simulink model "Octocopter2D_06States"  (R2018b)
settings: Solver=VariableStepAuto  StartTime=0.0  StopTime=10  MaxStep=1e-3  RelTol=1e-3
undefined symbols (not defined in the file): Uav
libraries: simulink_extras x3
settings Model: Creator=jeremie  LastModifiedBy=jban039
settings SFSimCC: SimUseLocalCustomCode=off
settings RTWCC: RTWUseLocalCustomCode=off

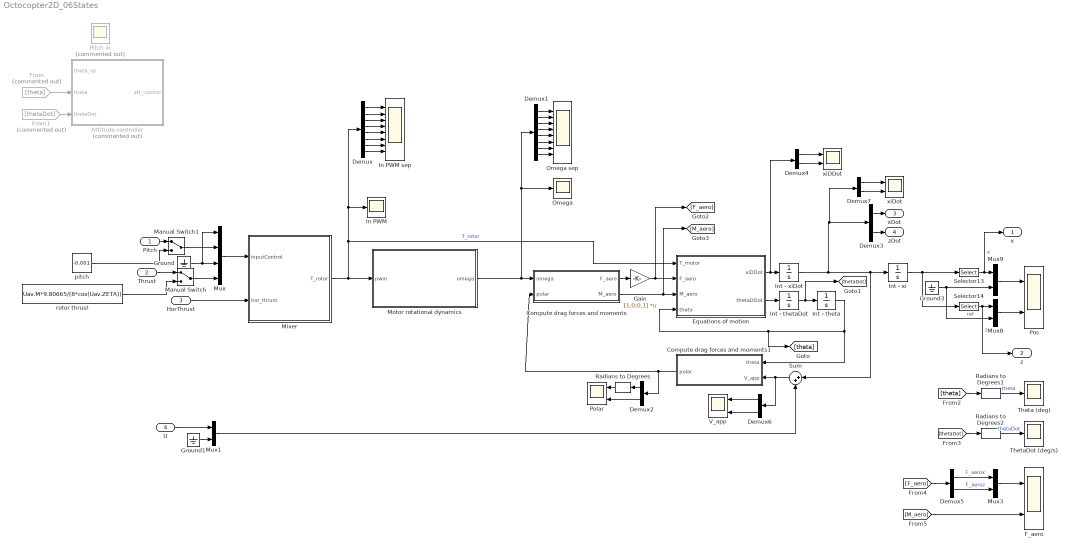
== system Octocopter2D_06States ==
  Pitch : Inport
  Thrust : Inport  Port=2
  HorThrust : Inport  Port=3
  U : Inport  Port=4
  Attitude controller : Subsystem  Commented=on
  Compute drag forces and moments : MATLAB Function  TreatAsAtomicUnit=on
  Compute drag forces and moments1 : MATLAB Function  TreatAsAtomicUnit=on
  Demux : Demux  Outputs=8
  Demux1 : Demux  Outputs=8
  Demux{2..7} (6 alike) : Demux  Outputs=2
  Equations of motion : MATLAB Function  TreatAsAtomicUnit=on
  F_aero : Scope  NumInputPorts=2
  From : From  Commented=on  GotoTag=theta
  From1 : From  Commented=on  GotoTag=thetaDot
  Gain : Gain  Gain=[1,0;0,1]  Multiplication=Matrix(K*u)
  Ground : Ground
  Ground1 : Ground
  Ground3 : Ground
  In PWM : Scope
  In PWM sep : Scope  NumInputPorts=8
  Int - theta : Integrator  ContinuousStateAttributes='theta'
  Int - thetaDot : Integrator  ContinuousStateAttributes='thetaDot'
  Int - xi : Integrator  ContinuousStateAttributes={'x','z'}
  Int - xiDot : Integrator  ContinuousStateAttributes={'xDot','zDot'}
  Manual Switch : ManualSwitch
  Manual Switch1 : ManualSwitch
  Mixer : MATLAB Function  TreatAsAtomicUnit=on
  Motor rotational dynamics : MATLAB Function  TreatAsAtomicUnit=on
  Mux : Mux
  Mux{1,3,8..9} (4 alike) : Mux  Inputs=2
  Omega : Scope
  Omega sep : Scope  NumInputPorts=8
  Pitch in : Scope  Commented=on
  Polar : Scope  NumInputPorts=2
  Pos : Scope  NumInputPorts=2
  Radians to Degrees : simulink_extras/Transformations/Radians to Degrees
  Radians to Degrees1 : simulink_extras/Transformations/Radians to Degrees
  Radians to Degrees2 : simulink_extras/Transformations/Radians to Degrees
  Selector13 : Selector  InputPortWidth=2  IndexOptions=Index vector (dialog)  Indices=1  OutputSizes=1
  Selector14 : Selector  InputPortWidth=2  IndexOptions=Index vector (dialog)  Indices=2  OutputSizes=1
  Sum : Sum  Inputs=|++
  Theta (deg) : Scope
  ThetaDot (deg/s) : Scope
  V_app : Scope  NumInputPorts=2
  pitch : Constant  Value=-0.001
  rotor thrust : Constant  Value=Uav.M*9.80665/(8*cos(Uav.ZETA))
  xiDDot : Scope  NumInputPorts=2
  xiDot : Scope  NumInputPorts=2
  x : Outport
  z : Outport  Port=2
  xDot : Outport  Port=3
  zDot : Outport  Port=4
  wires:
  Motor rotational dynamics/1(omega) -> Compute drag forces and moments/1(omega), Omega/1, Demux1/1
  Compute drag forces and moments/1(F_aero) -> Gain/1
  Compute drag forces and moments/2(M_aero) -> Equations of motion/3(M_aero), [M_aero]
  Mixer/1(T_rotor) -> Demux/1, In PWM/1, Equations of motion/1(T_motor), Motor rotational dynamics/1(pwm)  "T_rotor"
  Mux/1 -> Mixer/1(inputControl)
  Ground/1 -> Mux/3, Mux/1
  Manual Switch1/1 -> Mux/2
  Manual Switch/1 -> Mux/4
  Equations of motion/1(xiDDot) -> Demux4/1, Int - xiDot/1
  Equations of motion/2(thetaDDot) -> Int - thetaDot/1
  Int - thetaDot/1 -> [thetaDot], Int - theta/1
  Int - theta/1 -> [theta], Equations of motion/4(theta), Compute drag forces and moments1/1(theta)
  Mux1/1 -> Sum/2
  Sum/1 -> Demux6/1, Compute drag forces and moments1/2(V_app)
  Compute drag forces and moments1/1(polar) -> Demux2/1, Compute drag forces and moments/2(polar)
  Ground3/1 -> Mux8/2, Mux9/2  "ref"
  Selector14/1 -> z/1, Mux8/1  "z"
  Selector13/1 -> x/1, Mux9/1  "x"
  Mux8/1 -> Pos/2
  Mux9/1 -> Pos/1
  Int - xi/1 -> Selector14/1, Selector13/1
  Demux/1 -> In PWM sep/1
  Demux/2 -> In PWM sep/2
  Demux/3 -> In PWM sep/3
  Demux/4 -> In PWM sep/4
  Demux/5 -> In PWM sep/5
  Demux/6 -> In PWM sep/6
  Demux/7 -> In PWM sep/7
  Demux/8 -> In PWM sep/8
  Demux1/8 -> Omega sep/8
  Demux1/7 -> Omega sep/7
  Demux1/6 -> Omega sep/6
  Demux1/5 -> Omega sep/5
  Demux1/4 -> Omega sep/4
  Demux1/3 -> Omega sep/3
  Demux1/2 -> Omega sep/2
  Demux1/1 -> Omega sep/1
  Demux2/2 -> Polar/2
  Demux2/1 -> Radians to Degrees/1
  Radians to Degrees/1 -> Polar/1
  Radians to Degrees1/1 -> Theta (deg)/1  "theta"
  From/1 -> Attitude controller/2(theta)
  From1/1 -> Attitude controller/3(thetaDot)
  HorThrust/1 -> Mixer/2(hor_thrust)
  [theta] -> Radians to Degrees1/1
  Demux3/1 -> xDot/1
  Demux3/2 -> zDot/1
  Demux4/1 -> xiDDot/1
  Demux4/2 -> xiDDot/2
  [thetaDot] -> Radians to Degrees2/1
  Radians to Degrees2/1 -> ThetaDot (deg/s)/1  "thetaDot"
  U/1 -> Mux1/1
  Ground1/1 -> Mux1/2
  Mux3/1 -> F_aero/1
  [M_aero] -> F_aero/2
  Demux5/1 -> Mux3/1  "F_aerox"
  Demux5/2 -> Mux3/2  "F_aeroz"
  [F_aero] -> Demux5/1
  Thrust/1 -> Manual Switch/1
  rotor thrust/1 -> Manual Switch/2
  Pitch/1 -> Manual Switch1/1
  pitch/1 -> Manual Switch1/2
  Demux6/1 -> V_app/1
  Demux6/2 -> V_app/2
  Demux7/2 -> xiDot/2
  Demux7/1 -> xiDot/1
  Int - xiDot/1 -> Demux7/1, Demux3/1, Sum/1, Int - xi/1
  Gain/1 -> Equations of motion/2(F_aero), [F_aero]

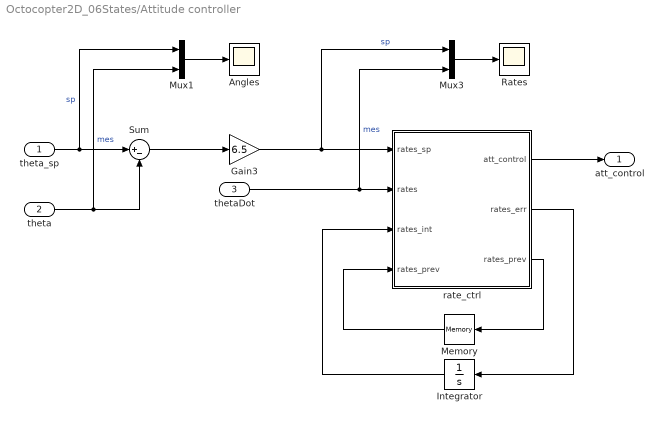
== system Octocopter2D_06States/Attitude controller ==
  theta_sp : Inport
  theta : Inport  Port=2
  thetaDot : Inport  Port=3
  Angles : Scope
  Gain3 : Gain  Gain=6.5
  Integrator : Integrator
  Memory : Memory
  Mux1 : Mux  Inputs=2
  Mux3 : Mux  Inputs=2
  Rates : Scope
  Sum : Sum  Inputs=|+-
  rate_ctrl : MATLAB Function  TreatAsAtomicUnit=on  SystemSampleTime=0.002
  att_control : Outport
  wires:
  rate_ctrl/2(rates_err) -> Integrator/1
  rate_ctrl/3(rates_prev) -> Memory/1
  Integrator/1 -> rate_ctrl/3(rates_int)
  rate_ctrl/1(att_control) -> att_control/1
  Memory/1 -> rate_ctrl/4("rates_prev ")
  Mux3/1 -> Rates/1
  thetaDot/1 -> rate_ctrl/2(rates), Mux3/2  "mes"
  Gain3/1 -> rate_ctrl/1(rates_sp), Mux3/1  "sp"
  Sum/1 -> Gain3/1
  theta_sp/1 -> Mux1/1, Sum/1  "sp"
  theta/1 -> Mux1/2, Sum/2  "mes"
  Mux1/1 -> Angles/1

== matlab function Octocopter2D_06States/Attitude controller/rate_ctrl ==
  data: rates_sp input size=1; rates input size=1; att_control output size=1; rates_err output; rates_prev output; rates_int input size=1; rates_prev input size=1
function [ att_control, rates_err, rates_prev ] = rate_ctrl(rates_sp, rates, rates_int, rates_prev)
rates_p = 0.15;
rates_i = 0.05;
rates_d = 0.003;
rate_ff = 0;

dt = 0.002;

% Angular rates error
rates_err = - rates_sp + rates;

% % Perform the integration using a first order method and do not propaate the result if out of range or invalid
% rates_int = rates_int +  rates_err * dt;

att_control = rates_p .* rates_err + rates_i .* rates_int + rates_d .* (rates_prev - rates) ./ dt + rate_ff .* rates_sp;

rates_prev = rates;

end

== matlab function Octocopter2D_06States/Compute drag forces and moments ==
  data: omega input; polar input size=2; F_aero output; M_aero output; Uav parameter
function [F_aero, M_aero] = computeAero( omega, polar, Uav )
%#codegen

% Name variables
alpha    = -polar(1); % equations assume alpha measured the other way
U        = polar(2);
omegaBar = mean(omega);
rho      = Uav.RHO_AIR;
D_UAV    = Uav.D_UAV;
A_UAV    = Uav.A_UAV;
D_PROP   = Uav.D_PROP;
A_PROP   = Uav.A_PROP;
n        = Uav.N_ROTORS;

% Force coefficients
Cxb1 = -0.241*cos(alpha) + 0.036*cos(3*alpha) + 0.016*cos(7*alpha);
Cxb2 = -0.053*cos(alpha) - 0.008*cos(3*alpha);
Czb1 = -0.724*sin(alpha) + 0.080;
Czb2 = -0.222*sin(alpha) + 0.065;

% Moment coefficients
lambda = omegaBar*D_PROP / ( 2*U );
A1  =  0.116 * ( 1 - exp(-0.126*lambda) );
A2  = -0.041 * ( 1 - exp(-0.308*lambda) );
CM1 =  0.009*cos(alpha) + 0.003*cos(3*alpha) - 0.014*sin(2*alpha);
CM2 =  A1*cos(alpha) + A2*sin(2*alpha);

% Forces and moments
Fxb = 0.5*rho*U^2*Cxb1*A_UAV      + 0.5*rho*U*omegaBar*Cxb2*D_PROP*A_PROP*(n/4);
Fzb = 0.5*rho*U^2*Czb1*A_UAV      + 0.5*rho*U*omegaBar*Czb2*D_PROP*A_PROP*(n/4);
M   = 0.5*rho*U^2*CM1*A_UAV*D_UAV + 0.5*rho*U*omegaBar*CM2*D_PROP^2*A_PROP*(n/4);

% Output forces - NED
F_aero = [ Fxb; -Fzb ];
M_aero = M;

== matlab function Octocopter2D_06States/Motor rotational dynamics ==
  data: pwm input; omega output; Uav parameter
function omega = motorRotDynamics( pwm, Uav )
%#codegen

omega = sqrt( abs(pwm)/(cos(Uav.ZETA)*Uav.C_T) );

== matlab function Octocopter2D_06States/Equations of motion ==
  data: T_motor input; xiDDot output; F_aero input size=2; M_aero input; theta input; thetaDDot output; Uav parameter
function [ xiDDot, thetaDDot ] = Octo2DModel( T_motor, F_aero, M_aero, theta, Uav )
%#codegen

% Name variables
m_UAV = Uav.M;
J_UAV = Uav.J;
D_UAV = Uav.D_UAV;
Fxb = F_aero(1);
Fzb = F_aero(2);
g = 9.80665;
zeta = Uav.ZETA;

% Forces and pitching moment in body frame
T   = -cos(zeta)*sum(T_motor);
Txb = 2*sin(zeta)*(T_motor(3) - T_motor(2));

M = cos(zeta)*D_UAV*( ...
    T_motor(1)*sind(22.5) + T_motor(2)*cosd(22.5) - ...
    T_motor(3)*cosd(22.5) - T_motor(4)*sind(22.5) );

% Forces and pitching moment in world frame
xDDot = ( (T + Fzb)*sin(theta) + (Txb + Fxb)*cos(theta) ) / m_UAV;
zDDot = ( (T + Fzb)*cos(theta) + (Txb + Fxb)*sin(theta) + m_UAV*g ) / m_UAV;

xiDDot = [xDDot; zDDot];
thetaDDot = (M + M_aero) / J_UAV;

end

== matlab function Octocopter2D_06States/Mixer ==
  data: inputControl input size=4; T_rotor output size=8; hor_thrust input
function T_rotor = mix( inputControl, hor_thrust )
%#codegen
    ROTOR_COUNT = 8;
    a = tand(22.5);

    % Motor map from Jeremy
    rotors = struct( 'roll_scale',   {-0.383,  0.383, -0.924, -0.383,  0.383,  0.924,  0.924, -0.924}, ...
                     'pitch_scale',  { 0.924, -0.924,  0.383, -0.924,  0.924, -0.383,  0.383, -0.383}, ...
                     'yaw_scale',    {-1, -1,  1,  1,  1,  1, -1, -1}, ...
                     'thrust_scale', { 1,  1,  1,  1,  1,  1,  1,  1}, ...
                     'hor_thrust_scale', {a*1,  -a*1,  -1,  -a*1,  a*1,  1,  -1,  1});

    roll   = inputControl(1);
    pitch  = inputControl(2);
    yaw    = inputControl(3);
    thrust = inputControl(4);
    outputControl = zeros(ROTOR_COUNT,1);

    % /* perform initial mix pass yielding unbounded outputs, ignore yaw */
    for i = 1:ROTOR_COUNT
        out = pitch * rotors(i).pitch_scale ...
              + thrust ...
              + hor_thrust*rotors(i).hor_thrust_scale;

        outputControl(i) = out;
    end
    T_rotor = [ outputControl(1);
                outputControl(3);
                outputControl(8);
                outputControl(4);
                outputControl(2);
                outputControl(6);
                outputControl(7);
                outputControl(5) ];
end

== matlab function Octocopter2D_06States/Compute drag forces and moments1 ==
  data: theta input; V_app input; polar output
function polar   = computeSph( theta, V_app )
%#codegen

V_appBody = [ cos(theta), -sin(theta); sin(theta), cos(theta) ] * V_app; % CHECK

% alpha = theta since wind is horizontal
polar = [atan2(V_appBody(2), V_appBody(1)); norm(V_appBody)];
